simulink model "EMT_load"  (R2024a)
settings: Solver=ode1  StartTime=0.0  StopTime=simtime  FixedStep=Ts  RelTol=1e-3
values from neighbouring files (symbols this model uses):
  c0 = c0_hawk    (= 6.37282e-09)    [EMT_Phasor_parameters.m]
  c1 = c1_hawk    (= 8.76156e-09)    [EMT_Phasor_parameters.m]
  fg = 50    [EMT_Phasor_parameters.m]
  G1gen = 0.1245    [EMT_Phasor_parameters.m]
  G2gen = 0.30    (= 0.3)    [EMT_Phasor_parameters.m]
  G3gen = 0.20    (= 0.2)    [EMT_Phasor_parameters.m]
  G4sgen = 0.2078    [EMT_Phasor_parameters.m]
  G5gen = 0.20    (= 0.2)    [EMT_Phasor_parameters.m]
  G6gen = 0.2078    [EMT_Phasor_parameters.m]
  G6sgen = 0.20    (= 0.2)    [EMT_Phasor_parameters.m]
  G7gen = 0.518    [EMT_Phasor_parameters.m]
  Ihvpk = Ihv*sqrt(2)    [EMT_Phasor_parameters.m]
  l0 = l0_hawk    (= 0.00373)    [EMT_Phasor_parameters.m]
  l1 = l1_hawk    (= 0.00133)    [EMT_Phasor_parameters.m]
  L3dem = 0.10    (= 0.1)    [EMT_Phasor_parameters.m]
  L4dem = 0.30    (= 0.3)    [EMT_Phasor_parameters.m]
  L5dem = 0.35    [EMT_Phasor_parameters.m]
  L6dem = 0.15    [EMT_Phasor_parameters.m]
  L7dem = 0.10    (= 0.1)    [EMT_Phasor_parameters.m]
  Pr = Sr*PF    (= 550050000)    [EMT_Phasor_parameters.m]
  Qr = sqrt(Sr^2 - Pr^2)    [EMT_Phasor_parameters.m]
  r0 = r0_hawk    (= 0.44587)    [EMT_Phasor_parameters.m]
  r1 = r1_hawk    (= 0.12087)    [EMT_Phasor_parameters.m]
  Rtpu = Xtpu/40    (= 0.00375)    [EMT_Phasor_parameters.m]
  S1non = 400e6    (= 400000000)    [EMT_Phasor_parameters.m]
  S2non = 300e6    (= 300000000)    [EMT_Phasor_parameters.m]
  S3non = 200e6    (= 200000000)    [EMT_Phasor_parameters.m]
  S4snon = 200e6    (= 200000000)    [EMT_Phasor_parameters.m]
  S5non = 500e6    (= 500000000)    [EMT_Phasor_parameters.m]
  S6non = 400e6    (= 400000000)    [EMT_Phasor_parameters.m]
  S6snon = 200e6    (= 200000000)    [EMT_Phasor_parameters.m]
  S7non = 200e6    (= 200000000)    [EMT_Phasor_parameters.m]
  simtime = 5    [EMT_Phasor_parameters.m]
  tonvsc = 0.01    [EMT_Phasor_parameters.m]
  Ts = 150e-6    (= 0.00015)    [EMT_Phasor_parameters.m]
  Vhv = 220e3    (= 220000)    [EMT_Phasor_parameters.m]
  Vmv = 22e3    (= 22000)    [EMT_Phasor_parameters.m]
  wc1 = wsw1/10    (= 848.230016469)    [EMT_Phasor_parameters.m]
  wdc1 = wc1/10    (= 84.8230016469)    [EMT_Phasor_parameters.m]
  wpq1 = wc1/10    (= 84.8230016469)    [EMT_Phasor_parameters.m]
  wsw1 = ksw1*2*pi*fg    (= 8482.30016469)    [EMT_Phasor_parameters.m]
  Xtpu = 0.15    [EMT_Phasor_parameters.m]
undefined symbols (not defined in the file or in its folder): D11, Delta, Kf, r, theta0
libraries: simulink_extras x152, spsGroundLib x49, spsCurrentMeasurementLib x39, spsVoltageMeasurementLib x33, simulink x32, eeGeneralControl x32, slpidlib x32, powerlib x30, powerlib_meascontrol x28, spsFirstOrderFilterLib x24, eeTransforms x24, pid_lib x16
(part 5 of 16)

== system EMT_load/G6/VSC/VI measurement ==
  Current Measurement : spsCurrentMeasurementLib/Current Measurement  PhasorSimulation=off  OutputType=Complex  PSBequivalent=0
  Current Measurement1 : spsCurrentMeasurementLib/Current Measurement  PhasorSimulation=off  OutputType=Complex  PSBequivalent=0
  Current Measurement2 : spsCurrentMeasurementLib/Current Measurement  PhasorSimulation=off  OutputType=Complex  PSBequivalent=0
  Ground : spsGroundLib/Ground  LConnTagsString=a
  Ground1 : spsGroundLib/Ground  LConnTagsString=a
  Ground2 : spsGroundLib/Ground  LConnTagsString=a
  Mux : Mux  Inputs=3
  Mux1 : Mux  Inputs=3
  Voltage Measurement : spsVoltageMeasurementLib/Voltage Measurement  PhasorSimulation=off  OutputType=Complex  PSBequivalent=0
  Voltage Measurement1 : spsVoltageMeasurementLib/Voltage Measurement  PhasorSimulation=off  OutputType=Complex  PSBequivalent=0
  Voltage Measurement2 : spsVoltageMeasurementLib/Voltage Measurement  PhasorSimulation=off  OutputType=Complex  PSBequivalent=0
  A : PMIOPort  Side=Left
  B : PMIOPort  Port=2  Side=Left
  C : PMIOPort  Port=3  Side=Left
  a : PMIOPort  Port=4  Side=Right
  b : PMIOPort  Port=5  Side=Right
  c : PMIOPort  Port=6  Side=Right
  Vs : Outport
  Is : Outport  Port=2
  wires:
  Mux1/1 -> Is/1
  Mux/1 -> Vs/1
  Voltage Measurement1/1 -> Mux/2
  Voltage Measurement2/1 -> Mux/3
  Current Measurement2/1 -> Mux1/3
  Voltage Measurement/1 -> Mux/1
  Current Measurement/1 -> Mux1/1
  Current Measurement1/1 -> Mux1/2
  connections:
  Voltage Measurement/LConn1 -- Current Measurement/LConn1 -- A/RConn1
  Current Measurement2/LConn1 -- C/RConn1 -- Voltage Measurement2/LConn1
  Current Measurement1/LConn1 -- Voltage Measurement1/LConn1 -- B/RConn1
  Current Measurement1/RConn1 -- b/RConn1
  Current Measurement/RConn1 -- a/RConn1
  Ground/LConn1 -- Voltage Measurement/LConn2
  Current Measurement2/RConn1 -- c/RConn1
  Ground1/LConn1 -- Voltage Measurement1/LConn2
  Ground2/LConn1 -- Voltage Measurement2/LConn2

== system EMT_load/G6/VSC/VSC Control ==
  Block : Inport
  Vabc : Inport  Port=2
  Iabc : Inport  Port=3
  Pset : Inport  Port=4
  Qset : Inport  Port=5
  Control loops : Subsystem  Variant=on  VariantControlMode=label  LabelModeActiveChoice=EMT_and_QEMT
  Measurements : Subsystem  Variant=on  VariantControlMode=label  LabelModeActiveChoice=EMT
  Modulation : Subsystem  Variant=on  VariantControlMode=label  LabelModeActiveChoice=EMT_AVG
  Mux : Mux  Inputs=2
  Ref : Outport
  m : Outport  Port=2
  wires:
  Control loops/2(iqd+-ref) -> Modulation/3(iqd+-*)
  Control loops/1(vqd+-ref) -> Modulation/2(vqd+-*)
  [PQabc] -> Mux/2
  Measurements/5(PQabc) -> [PQabc]
  Modulation/1(Ref) -> Ref/1
  Measurements/4(theta) -> [theta]
  Vabc/1 -> Measurements/1(Vabc)
  Measurements/1(vqd+-) -> Control loops/3(vqd+-), [vqdpn]
  Measurements/2(iqd+-) -> Control loops/4(iqd+-)
  Measurements/3(freq) -> Control loops/5(freq)
  [theta] -> Modulation/4(theta)
  [vqdpn] -> Modulation/1(vqd+-)
  Iabc/1 -> Measurements/2(Iabc)
  Mux/1 -> m/1
  Control loops/3(m) -> Mux/1
  Pset/1 -> Control loops/1(Pset)
  Qset/1 -> Control loops/2(Qset)
  Block/1 -> Control loops/6(Block)

== system EMT_load/G6/VSC/VSC Model ==
  Ref : Inport
  EMT AVG : Subsystem  VariantControl=EMT_AVG
      settings: PortSchema="{\"entries\":[{\"content\":{\"sides\":[{\"content\":{\"connectorIds\":[\"LConn1\",\"LConn2\",\"LConn3\"]},\"type\":\"ConnectorPlacement.EquallySpacedRectSide\",\"uuid\":\"96043b84-a665-4cb2-a938-d6633d7ee474\"},{\"content\":{\"connectorIds\":[\"In1\"],\"side\":\"RIGHT\"},\"type\":\"ConnectorPlacement.EquallySpacedRectSide\",\"uuid\":\"064d463f-c23a-42ac-89ce-8dea3d446214\"},{\"content\":{\"connectorIds\":[],\"side\":\"TOP\"},\"type\":\"ConnectorPlacement.EquallySpacedRectSide\",\"uuid\":\"95ef669c-c6ed-44c3-8b69-447906728b6d\"}]},\"type\":\"ConnectorPlacement.EquallySpacedConnector\",\"uuid\":\"ea66db09-64d7-4d7e-ba7b-d769c56e2dbd\"}],\"packageUris\":[\"http://schema.mathworks.com/mf0/Connector/19700101\"],\"version\":\"1.0\"}"
  EMT SW : Subsystem  VariantControl=EMT_SW
      settings: PortSchema="{\"entries\":[{\"content\":{\"sides\":[{\"content\":{\"connectorIds\":[\"LConn1\",\"LConn2\",\"LConn3\"]},\"type\":\"ConnectorPlacement.EquallySpacedRectSide\",\"uuid\":\"96043b84-a665-4cb2-a938-d6633d7ee474\"},{\"content\":{\"connectorIds\":[\"In1\"],\"side\":\"RIGHT\"},\"type\":\"ConnectorPlacement.EquallySpacedRectSide\",\"uuid\":\"064d463f-c23a-42ac-89ce-8dea3d446214\"},{\"content\":{\"connectorIds\":[],\"side\":\"TOP\"},\"type\":\"ConnectorPlacement.EquallySpacedRectSide\",\"uuid\":\"95ef669c-c6ed-44c3-8b69-447906728b6d\"}]},\"type\":\"ConnectorPlacement.EquallySpacedConnector\",\"uuid\":\"ea66db09-64d7-4d7e-ba7b-d769c56e2dbd\"}],\"packageUris\":[\"http://schema.mathworks.com/mf0/Connector/19700101\"],\"version\":\"1.0\"}"
  Phasor : Subsystem  VariantControl=Phasor
      settings: PortSchema="{\"entries\":[{\"content\":{\"sides\":[{\"content\":{\"connectorIds\":[\"LConn1\",\"LConn2\",\"LConn3\"]},\"type\":\"ConnectorPlacement.EquallySpacedRectSide\",\"uuid\":\"96043b84-a665-4cb2-a938-d6633d7ee474\"},{\"content\":{\"connectorIds\":[\"In1\"],\"side\":\"RIGHT\"},\"type\":\"ConnectorPlacement.EquallySpacedRectSide\",\"uuid\":\"064d463f-c23a-42ac-89ce-8dea3d446214\"},{\"content\":{\"connectorIds\":[],\"side\":\"TOP\"},\"type\":\"ConnectorPlacement.EquallySpacedRectSide\",\"uuid\":\"95ef669c-c6ed-44c3-8b69-447906728b6d\"}]},\"type\":\"ConnectorPlacement.EquallySpacedConnector\",\"uuid\":\"ea66db09-64d7-4d7e-ba7b-d769c56e2dbd\"}],\"packageUris\":[\"http://schema.mathworks.com/mf0/Connector/19700101\"],\"version\":\"1.0\"}"
  A : PMIOPort  Side=Left
  B : PMIOPort  Port=2  Side=Left
  C : PMIOPort  Port=3  Side=Left

== system EMT_load/G6/VSC/output signals ==
  Vs : Inport
  Is : Inport  Port=2
  control : Inport  Port=3
  Bus Creator : BusCreator  Inputs=15
  Demux : Demux  Outputs=13
  m : Outport
  wires:
  Bus Creator/1 -> m/1
  control/1 -> Demux/1
  Vs/1 -> Bus Creator/1  "Vabc"
  Is/1 -> Bus Creator/2  "Iabc"
  Demux/1 -> Bus Creator/3  "vqp"
  Demux/2 -> Bus Creator/4  "vdp"
  Demux/3 -> Bus Creator/5  "vqn"
  Demux/4 -> Bus Creator/6  "vdn"
  Demux/5 -> Bus Creator/7  "iqp"
  Demux/6 -> Bus Creator/8  "idp"
  Demux/7 -> Bus Creator/9  "iqn"
  Demux/8 -> Bus Creator/10  "idn"
  Demux/9 -> Bus Creator/11  "f"
  Demux/10 -> Bus Creator/12  "Pdq"
  Demux/11 -> Bus Creator/13  "Qdq"
  Demux/12 -> Bus Creator/14  "Pabc"
  Demux/13 -> Bus Creator/15  "Qabc"

== system EMT_load/G6s/Exciter System/PSS ==
  note: Power System Stabilizer (PSS2A)
  dw : Inport
  Pgen : Inport  Port=2
  Gain : Gain  Gain=Ks1
  Gain1 : Gain  Gain=Ks3
  Saturation : Saturate  UpperLimit=Vstmax  LowerLimit=Vstmin
  Sum1 : Sum  Inputs=|++
  Sum2 : Sum  Inputs=|+-
  Transfer Fcn1 : TransferFcn  Numerator=[Tw1 0]  Denominator=[Tw1 1]
  Transfer Fcn2 : TransferFcn  Numerator=[Tw3 0]  Denominator=[Tw3 1]
  Transfer Fcn3 : TransferFcn  Numerator=[Tw2 0]  Denominator=[Tw2 1]
  Transfer Fcn4 : TransferFcn  Denominator=[T6 1]
  Transfer Fcn5 : TransferFcn  Numerator=[T8 1].^N  Denominator=[T9 1].^(M*N)
  Transfer Fcn6 : TransferFcn  Numerator=[T1 1]  Denominator=[T2 1]
  Transfer Fcn7 : TransferFcn  Numerator=[T3 1]  Denominator=[T4 1]
  Transfer Fcn8 : TransferFcn  Numerator=[Tw4 0]  Denominator=[Tw4 1]
  Transfer Fcn9 : TransferFcn  Numerator=[Ks2]  Denominator=[T7 1]
  Vothsg : Outport
  wires:
  Transfer Fcn9/1 -> Sum2/2, Gain1/1
  Gain1/1 -> Sum1/2
  Transfer Fcn8/1 -> Transfer Fcn9/1
  Transfer Fcn2/1 -> Transfer Fcn8/1
  Pgen/1 -> Transfer Fcn2/1
  Saturation/1 -> Vothsg/1
  Transfer Fcn7/1 -> Saturation/1
  Transfer Fcn6/1 -> Transfer Fcn7/1
  Gain/1 -> Transfer Fcn6/1
  Sum2/1 -> Gain/1
  Transfer Fcn5/1 -> Sum2/1
  Sum1/1 -> Transfer Fcn5/1
  Transfer Fcn4/1 -> Sum1/1
  Transfer Fcn3/1 -> Transfer Fcn4/1
  Transfer Fcn1/1 -> Transfer Fcn3/1
  dw/1 -> Transfer Fcn1/1

== system EMT_load/G6s/Exciter System/SEXS ==
  note: The controller parameters provided by ENTSO-E
      | define different names for the parameters:
      |
      | ENTSO-E = IEEE Std 421.5-2005
      | Ta = Tc
      | Tb = Tb
      | K = Ka
      | Te = Ta
      | Emax = Vrmax
      | Emin = Vrmin
  note: The exciter model provided by ENTSO-E most similar to the IEEE is the Type AC4A excitation system model
  Vref : Inport
  Vc : Inport  Port=2
  Vs : Inport  Port=3
  1st ord transfer fcn windup limiter : Subsystem  mask{Gain=K, tau=Te, Vmax=Emax, Vmin=Emin, y0=Vf0}
      mask prompts: tau "Time constant"; y0 "Initial output"
  Constant : Constant  Value=Vf0/K
  Saturation : Saturate  Commented=through  UpperLimit=0.1  LowerLimit=-0.1
  Sum : Sum  Inputs=+-+
  Sum1 : Sum  Inputs=|++
  Transfer Fcn (with initial outputs)1 : simulink_extras/Additional Linear/Transfer Fcn (with initial outputs)  N=[Ta 1]  D=[Tb 1]  Y0=Vf0/K  U0=Vf0/K
  Efd : Outport
  wires:
  1st ord transfer fcn windup limiter/1(Out1) -> Efd/1
  Vs/1 -> Sum/3
  Vref/1 -> Sum/1
  Vc/1 -> Sum/2
  Transfer Fcn (with initial outputs)1/1 -> 1st ord transfer fcn windup limiter/1(In1)
  Saturation/1 -> Transfer Fcn (with initial outputs)1/1
  Sum/1 -> Sum1/1
  Sum1/1 -> Saturation/1
  Constant/1 -> Sum1/2

== system EMT_load/G6s/Exciter System/TR and LC_test ==
  note: Rc and Xc should be negative values in case of voltage regulated after an impedance
  note: Fig 4.1 of IEEE Std 421.5-2005
  note: Vt and It should be phasors (complex quantities)
  note: compensated
      | impedance
  note: Terminal voltage transducer and optional load compensation
  Vt : Inport
  It : Inport  Port=2
  Abs : Abs  SaturateOnIntegerOverflow=off
  Abs1 : Abs  SaturateOnIntegerOverflow=off
  Rc+jXc : Gain  Gain=abs(Rc+1i*Xc)
  Saturation : Saturate  UpperLimit=1.2  LowerLimit=0.8
  Sum : Sum  Inputs=|+-
  Transfer Fcn (with initial outputs) : simulink_extras/Additional Linear/Transfer Fcn (with initial outputs)  N=[1]  D=[Tr 1]  Y0=1  U0=1
  Vc : Outport
  wires:
  Abs1/1 -> Rc+jXc/1
  Abs/1 -> Sum/1
  It/1 -> Abs1/1
  Sum/1 -> Transfer Fcn (with initial outputs)/1
  Rc+jXc/1 -> Sum/2
  Transfer Fcn (with initial outputs)/1 -> Saturation/1
  Vt/1 -> Abs/1
  Saturation/1 -> Vc/1

== system EMT_load/G7/Exciter System/PSS1 ==
  note: Power System Stabilizer (PSS2A)
  dw : Inport
  Pgen : Inport  Port=2
  Gain : Gain  Gain=Ks1
  Gain1 : Gain  Gain=Ks3
  Saturation : Saturate  UpperLimit=Vstmax  LowerLimit=Vstmin
  Sum1 : Sum  Inputs=|++
  Sum2 : Sum  Inputs=|+-
  Transfer Fcn1 : TransferFcn  Numerator=[Tw1 0]  Denominator=[Tw1 1]
  Transfer Fcn2 : TransferFcn  Numerator=[Tw3 0]  Denominator=[Tw3 1]
  Transfer Fcn3 : TransferFcn  Numerator=[Tw2 0]  Denominator=[Tw2 1]
  Transfer Fcn4 : TransferFcn  Denominator=[T6 1]
  Transfer Fcn5 : TransferFcn  Numerator=[T8 1].^N  Denominator=[T9 1].^(M*N)
  Transfer Fcn6 : TransferFcn  Numerator=[T1 1]  Denominator=[T2 1]
  Transfer Fcn7 : TransferFcn  Numerator=[T3 1]  Denominator=[T4 1]
  Transfer Fcn8 : TransferFcn  Numerator=[Tw4 0]  Denominator=[Tw4 1]
  Transfer Fcn9 : TransferFcn  Numerator=[Ks2]  Denominator=[T7 1]
  Vothsg : Outport
  wires:
  dw/1 -> Transfer Fcn1/1
  Transfer Fcn1/1 -> Transfer Fcn3/1
  Transfer Fcn3/1 -> Transfer Fcn4/1
  Transfer Fcn4/1 -> Sum1/1
  Sum1/1 -> Transfer Fcn5/1
  Transfer Fcn5/1 -> Sum2/1
  Sum2/1 -> Gain/1
  Gain/1 -> Transfer Fcn6/1
  Transfer Fcn6/1 -> Transfer Fcn7/1
  Transfer Fcn7/1 -> Saturation/1
  Saturation/1 -> Vothsg/1
  Pgen/1 -> Transfer Fcn2/1
  Transfer Fcn2/1 -> Transfer Fcn8/1
  Transfer Fcn8/1 -> Transfer Fcn9/1
  Gain1/1 -> Sum1/2
  Transfer Fcn9/1 -> Gain1/1, Sum2/2

== system EMT_load/G7/Exciter System/SEXS ==
  note: The controller parameters provided by ENTSO-E
      | define different names for the parameters:
      |
      | ENTSO-E = IEEE Std 421.5-2005
      | Ta = Tc
      | Tb = Tb
      | K = Ka
      | Te = Ta
      | Emax = Vrmax
      | Emin = Vrmin
  note: The exciter model provided by ENTSO-E most similar to the IEEE is the Type AC4A excitation system model
  Vref : Inport
  Vc : Inport  Port=2
  Vs : Inport  Port=3
  1st ord transfer fcn windup limiter : Subsystem  mask{Gain=K, tau=Te, Vmax=Emax, Vmin=Emin, y0=Vf0}
      mask prompts: tau "Time constant"; y0 "Initial output"
  Constant : Constant  Value=Vf0/K
  Saturation : Saturate  Commented=through  UpperLimit=0.1  LowerLimit=-0.1
  Sum : Sum  Inputs=+-+
  Sum1 : Sum  Inputs=|++
  Transfer Fcn (with initial outputs)1 : simulink_extras/Additional Linear/Transfer Fcn (with initial outputs)  N=[Ta 1]  D=[Tb 1]  Y0=Vf0/K  U0=Vf0/K
  Efd : Outport
  wires:
  1st ord transfer fcn windup limiter/1(Out1) -> Efd/1
  Vs/1 -> Sum/3
  Vref/1 -> Sum/1
  Vc/1 -> Sum/2
  Transfer Fcn (with initial outputs)1/1 -> 1st ord transfer fcn windup limiter/1(In1)
  Saturation/1 -> Transfer Fcn (with initial outputs)1/1
  Sum/1 -> Sum1/1
  Sum1/1 -> Saturation/1
  Constant/1 -> Sum1/2

== system EMT_load/G7/Exciter System/TR and LC_test ==
  note: Terminal voltage transducer and optional load compensation
  note: compensated
      | impedance
  note: Vt and It should be phasors (complex quantities)
  note: Fig 4.1 of IEEE Std 421.5-2005
  note: Rc and Xc should be negative values in case of voltage regulated after an impedance
  Vt : Inport
  It : Inport  Port=2
  Abs : Abs  SaturateOnIntegerOverflow=off
  Abs1 : Abs  SaturateOnIntegerOverflow=off
  Rc+jXc : Gain  Gain=abs(Rc+1i*Xc)
  Saturation : Saturate  UpperLimit=1.2  LowerLimit=0.8
  Sum : Sum  Inputs=|+-
  Transfer Fcn (with initial outputs) : simulink_extras/Additional Linear/Transfer Fcn (with initial outputs)  Commented=through  N=[1]  D=[Tr 1]  Y0=1  U0=1
  Vc : Outport
  wires:
  Saturation/1 -> Vc/1
  Vt/1 -> Abs/1
  Transfer Fcn (with initial outputs)/1 -> Saturation/1
  Rc+jXc/1 -> Sum/2
  Sum/1 -> Transfer Fcn (with initial outputs)/1
  It/1 -> Abs1/1
  Abs/1 -> Sum/1
  Abs1/1 -> Rc+jXc/1

== system EMT_load/G1/Exciter System/SEXS/1st ord transfer fcn windup limiter ==
  note: First order transfer function with windup limiter (non-saturated output)
  In1 : Inport
  Compare To Constant : simulink/Logic and Bit Operations/Compare To Constant  relop=<=  const=Vmax  OutDataTypeStr=boolean
  Compare To Constant1 : simulink/Logic and Bit Operations/Compare To Constant  relop=>=  const=Vmin  OutDataTypeStr=boolean
  OR : Logic  Operator=OR  IconShape=distinctive  AllPortsSameDT=off  OutDataTypeStr=boolean
  Sample and Hold1 : spsSampleandHoldLib/Sample and Hold  ic=0  Ts=0
      settings: LibrarySourceBlock=|
      | sps_lib/Control/Sample and
      | Hold
  Saturation1 : Saturate  UpperLimit=Vmax  LowerLimit=Vmin
  Transfer Fcn (with initial outputs)2 : simulink_extras/Additional Linear/Transfer Fcn (with initial outputs)  N=[Gain]  D=[tau 1]  Y0=y0  U0=y0/Gain
  Out1 : Outport
  wires:
  Sample and Hold1/1 -> Transfer Fcn (with initial outputs)2/1
  Transfer Fcn (with initial outputs)2/1 -> Saturation1/1, Compare To Constant1/1, Compare To Constant/1
  In1/1 -> Sample and Hold1/1
  Compare To Constant/1 -> OR/1
  Compare To Constant1/1 -> OR/2
  OR/1 -> Sample and Hold1/2
  Saturation1/1 -> Out1/1

== system EMT_load/G2/VSC/VSC Control/Control loops ==
  note: 1) Add Subsystem or Model blocks as valid variant choices.
      | 2) You cannot connect blocks at this level. At simulation, connectivity is automatically
      | determined, based on the active variant and port name matching.
  Pset : Inport
  Qset : Inport  Port=2
  vqd+- : Inport  Port=3
  iqd+- : Inport  Port=4
  freq : Inport  Port=5
  Block : Inport  Port=6
  Phasor I 1st : Subsystem  VariantControl=Phasor_I_1st
  Phasor I ref : Subsystem  VariantControl=Phasor_I_ref
  Phasor PQ 1st : Subsystem  VariantControl=Phasor_PQ
  "SW, EMT AVG, Phasor Quasi-EMT" : Subsystem  VariantControl=EMT_and_QEMT
  vqd+-ref : Outport
  iqd+-ref : Outport  Port=2
  m : Outport  Port=3

== system EMT_load/G2/VSC/VSC Control/Measurements ==
  note: 1) Add Subsystem or Model blocks as valid variant choices.
      | 2) You cannot connect blocks at this level. At simulation, connectivity is automatically
      | determined, based on the active variant and port name matching.
  Vabc : Inport
  Iabc : Inport  Port=2
  EMT : Subsystem  VariantControl=EMT
  Phasor : Subsystem  VariantControl=Phasor
  vqd+- : Outport
  iqd+- : Outport  Port=2
  freq : Outport  Port=3
  theta : Outport  Port=4
  PQabc : Outport  Port=5

== system EMT_load/G2/VSC/VSC Control/Modulation ==
  note: 1) Add Subsystem or Model blocks as valid variant choices.
      | 2) You cannot connect blocks at this level. At simulation, connectivity is automatically
      | determined, based on the active variant and port name matching.
  vqd+- : Inport
  vqd+-* : Inport  Port=2
  iqd+-* : Inport  Port=3
  theta : Inport  Port=4
  EMT AVG : Subsystem  VariantControl=EMT_AVG
  EMT Switching : Subsystem  VariantControl=EMT_SW
  Phasor I and Phasor PQ : Subsystem  VariantControl=Phasor_I_and_PQ
  Phasor Quasi-EMT : Subsystem  VariantControl=Phasor_QEMT
  Ref : Outport

== system EMT_load/G2/VSC/VSC Model/EMT AVG ==
  Ref : Inport
  Controlled Voltage Source3 : spsControlledVoltageSourceLib/Controlled Voltage Source  Initialize=off  Source_Type=AC  Amplitude=Vhvpk  Phase=0  Frequency=fg  Measurements=None
  Controlled Voltage Source4 : spsControlledVoltageSourceLib/Controlled Voltage Source  Initialize=off  Source_Type=AC  Amplitude=Vhvpk  Phase=-2*pi/3  Frequency=fg  Measurements=None
  Controlled Voltage Source5 : spsControlledVoltageSourceLib/Controlled Voltage Source  Initialize=off  Source_Type=AC  Amplitude=Vhvpk  Phase=-4*pi/3  Frequency=fg  Measurements=None
  Demux1 : Demux  Outputs=3
  Ground : spsGroundLib/Ground  LConnTagsString=a
  Ground4 : spsGroundLib/Ground  LConnTagsString=a
  Ground5 : spsGroundLib/Ground  LConnTagsString=a
  A : PMIOPort  Side=Left
  B : PMIOPort  Port=2  Side=Left
  C : PMIOPort  Port=3  Side=Left
  wires:
  Ref/1 -> Demux1/1
  Demux1/1 -> Controlled Voltage Source3/1
  Demux1/2 -> Controlled Voltage Source4/1
  Demux1/3 -> Controlled Voltage Source5/1
  connections:
  Controlled Voltage Source3/RConn1 -- A/RConn1
  Controlled Voltage Source4/RConn1 -- B/RConn1
  Controlled Voltage Source5/RConn1 -- C/RConn1
  Ground/LConn1 -- Controlled Voltage Source3/LConn1
  Ground4/LConn1 -- Controlled Voltage Source4/LConn1
  Ground5/LConn1 -- Controlled Voltage Source5/LConn1

== system EMT_load/G2/VSC/VSC Model/EMT SW ==
  Ref : Inport
  DC Voltage Source : powerlib/Electrical Sources/DC Voltage Source  Amplitude=Vdc  Measurements=None
  Universal Bridge : powerlib/Power Electronics/Universal Bridge  Arms=3  SnubberResistance=1e6  SnubberCapacitance=inf  Device=IGBT / Diodes  Ron=1e-4  Lon=0  ForwardVoltages="[  0  0  ]"  ForwardVoltage=0  GTOparameters=[ 10e-6 , 20e-6 ]  IGBTparameters=[ 1e-6 , 2e-6 ]  Measurements=None  Measurements_2=None  converterType=Rectifier
  A : PMIOPort  Side=Left
  B : PMIOPort  Port=2  Side=Left
  C : PMIOPort  Port=3  Side=Left
  wires:
  Ref/1 -> Universal Bridge/1
  connections:
  Universal Bridge/LConn2 -- B/RConn1
  Universal Bridge/LConn1 -- A/RConn1
  Universal Bridge/LConn3 -- C/RConn1
  Universal Bridge/RConn1 -- DC Voltage Source/RConn1
  Universal Bridge/RConn2 -- DC Voltage Source/LConn1

== system EMT_load/G2/VSC/VSC Model/Phasor ==
  Ref : Inport
  Controlled Current Source : powerlib/Electrical Sources/Controlled Current Source  Initialize=off  Source_Type=AC  Amplitude=0  Phase=0  Frequency=0  Measurements=None
  Controlled Current Source1 : powerlib/Electrical Sources/Controlled Current Source  Initialize=off  Source_Type=AC  Amplitude=0  Phase=0  Frequency=0  Measurements=None
  Controlled Current Source2 : powerlib/Electrical Sources/Controlled Current Source  Initialize=off  Source_Type=AC  Amplitude=0  Phase=0  Frequency=0  Measurements=None
  Demux1 : Demux  Outputs=3
  Ground{1..3,5} (4 alike) : powerlib/Elements/Ground  LConnTagsString=a
  Three-Phase Series RLC Branch : powerlib/Elements/Three-Phase Series RLC Branch  LConnTagsString=A|B|C  RConnTagsString=A|B|C  BranchType=R  Resistance=1e7  Inductance=1e-3  Capacitance=1e-6  Measurements=None
  A : PMIOPort  Side=Left
  B : PMIOPort  Port=2  Side=Left
  C : PMIOPort  Port=3  Side=Left
  wires:
  [c] -> Controlled Current Source2/1
  [b] -> Controlled Current Source1/1
  [a] -> Controlled Current Source/1
  Demux1/3 -> [c]
  Demux1/2 -> [b]
  Demux1/1 -> [a]
  Ref/1 -> Demux1/1
  connections:
  Controlled Current Source/RConn1 -- Ground1/LConn1
  Controlled Current Source1/RConn1 -- Ground2/LConn1
  Controlled Current Source2/RConn1 -- Ground3/LConn1
  A/RConn1 -- Controlled Current Source/LConn1 -- Three-Phase Series RLC Branch/LConn1
  C/RConn1 -- Controlled Current Source2/LConn1 -- Three-Phase Series RLC Branch/LConn3
  Ground5/LConn1 -- Three-Phase Series RLC Branch/RConn2 -- Three-Phase Series RLC Branch/RConn1 -- Three-Phase Series RLC Branch/RConn3
  Controlled Current Source1/LConn1 -- Three-Phase Series RLC Branch/LConn2 -- B/RConn1

== system EMT_load/G3/VSC/VSC Control/Control loops ==
  note: 1) Add Subsystem or Model blocks as valid variant choices.
      | 2) You cannot connect blocks at this level. At simulation, connectivity is automatically
      | determined, based on the active variant and port name matching.
  Pset : Inport
  Qset : Inport  Port=2
  vqd+- : Inport  Port=3
  iqd+- : Inport  Port=4
  freq : Inport  Port=5
  Block : Inport  Port=6
  Phasor I 1st : Subsystem  VariantControl=Phasor_I_1st
  Phasor I ref : Subsystem  VariantControl=Phasor_I_ref
  Phasor PQ 1st : Subsystem  VariantControl=Phasor_PQ
  "SW, EMT AVG, Phasor Quasi-EMT" : Subsystem  VariantControl=EMT_and_QEMT
  vqd+-ref : Outport
  iqd+-ref : Outport  Port=2
  m : Outport  Port=3

== system EMT_load/G3/VSC/VSC Control/Measurements ==
  note: 1) Add Subsystem or Model blocks as valid variant choices.
      | 2) You cannot connect blocks at this level. At simulation, connectivity is automatically
      | determined, based on the active variant and port name matching.
  Vabc : Inport
  Iabc : Inport  Port=2
  EMT : Subsystem  VariantControl=EMT
  Phasor : Subsystem  VariantControl=Phasor
  vqd+- : Outport
  iqd+- : Outport  Port=2
  freq : Outport  Port=3
  theta : Outport  Port=4
  PQabc : Outport  Port=5

== system EMT_load/G3/VSC/VSC Control/Modulation ==
  note: 1) Add Subsystem or Model blocks as valid variant choices.
      | 2) You cannot connect blocks at this level. At simulation, connectivity is automatically
      | determined, based on the active variant and port name matching.
  vqd+- : Inport
  vqd+-* : Inport  Port=2
  iqd+-* : Inport  Port=3
  theta : Inport  Port=4
  EMT AVG : Subsystem  VariantControl=EMT_AVG
  EMT Switching : Subsystem  VariantControl=EMT_SW
  Phasor I and Phasor PQ : Subsystem  VariantControl=Phasor_I_and_PQ
  Phasor Quasi-EMT : Subsystem  VariantControl=Phasor_QEMT
  Ref : Outport

== system EMT_load/G3/VSC/VSC Model/EMT AVG ==
  Ref : Inport
  Controlled Voltage Source3 : spsControlledVoltageSourceLib/Controlled Voltage Source  Initialize=off  Source_Type=AC  Amplitude=Vhvpk  Phase=0  Frequency=fg  Measurements=None
  Controlled Voltage Source4 : spsControlledVoltageSourceLib/Controlled Voltage Source  Initialize=off  Source_Type=AC  Amplitude=Vhvpk  Phase=-2*pi/3  Frequency=fg  Measurements=None
  Controlled Voltage Source5 : spsControlledVoltageSourceLib/Controlled Voltage Source  Initialize=off  Source_Type=AC  Amplitude=Vhvpk  Phase=-4*pi/3  Frequency=fg  Measurements=None
  Demux1 : Demux  Outputs=3
  Ground : spsGroundLib/Ground  LConnTagsString=a
  Ground4 : spsGroundLib/Ground  LConnTagsString=a
  Ground5 : spsGroundLib/Ground  LConnTagsString=a
  A : PMIOPort  Side=Left
  B : PMIOPort  Port=2  Side=Left
  C : PMIOPort  Port=3  Side=Left
  wires:
  Ref/1 -> Demux1/1
  Demux1/1 -> Controlled Voltage Source3/1
  Demux1/2 -> Controlled Voltage Source4/1
  Demux1/3 -> Controlled Voltage Source5/1
  connections:
  Controlled Voltage Source3/RConn1 -- A/RConn1
  Controlled Voltage Source4/RConn1 -- B/RConn1
  Controlled Voltage Source5/RConn1 -- C/RConn1
  Ground/LConn1 -- Controlled Voltage Source3/LConn1
  Ground4/LConn1 -- Controlled Voltage Source4/LConn1
  Ground5/LConn1 -- Controlled Voltage Source5/LConn1

== system EMT_load/G3/VSC/VSC Model/EMT SW ==
  Ref : Inport
  DC Voltage Source : powerlib/Electrical Sources/DC Voltage Source  Amplitude=Vdc  Measurements=None
  Universal Bridge : powerlib/Power Electronics/Universal Bridge  Arms=3  SnubberResistance=1e6  SnubberCapacitance=inf  Device=IGBT / Diodes  Ron=1e-4  Lon=0  ForwardVoltages="[  0  0  ]"  ForwardVoltage=0  GTOparameters=[ 10e-6 , 20e-6 ]  IGBTparameters=[ 1e-6 , 2e-6 ]  Measurements=None  Measurements_2=None  converterType=Rectifier
  A : PMIOPort  Side=Left
  B : PMIOPort  Port=2  Side=Left
  C : PMIOPort  Port=3  Side=Left
  wires:
  Ref/1 -> Universal Bridge/1
  connections:
  Universal Bridge/LConn2 -- B/RConn1
  Universal Bridge/LConn1 -- A/RConn1
  Universal Bridge/LConn3 -- C/RConn1
  Universal Bridge/RConn1 -- DC Voltage Source/RConn1
  Universal Bridge/RConn2 -- DC Voltage Source/LConn1

== system EMT_load/G3/VSC/VSC Model/Phasor ==
  Ref : Inport
  Controlled Current Source : powerlib/Electrical Sources/Controlled Current Source  Initialize=off  Source_Type=AC  Amplitude=0  Phase=0  Frequency=0  Measurements=None
  Controlled Current Source1 : powerlib/Electrical Sources/Controlled Current Source  Initialize=off  Source_Type=AC  Amplitude=0  Phase=0  Frequency=0  Measurements=None
  Controlled Current Source2 : powerlib/Electrical Sources/Controlled Current Source  Initialize=off  Source_Type=AC  Amplitude=0  Phase=0  Frequency=0  Measurements=None
  Demux1 : Demux  Outputs=3
  Ground{1..3,5} (4 alike) : powerlib/Elements/Ground  LConnTagsString=a
  Three-Phase Series RLC Branch : powerlib/Elements/Three-Phase Series RLC Branch  LConnTagsString=A|B|C  RConnTagsString=A|B|C  BranchType=R  Resistance=1e7  Inductance=1e-3  Capacitance=1e-6  Measurements=None
  A : PMIOPort  Side=Left
  B : PMIOPort  Port=2  Side=Left
  C : PMIOPort  Port=3  Side=Left
  wires:
  [c] -> Controlled Current Source2/1
  [b] -> Controlled Current Source1/1
  [a] -> Controlled Current Source/1
  Demux1/3 -> [c]
  Demux1/2 -> [b]
  Demux1/1 -> [a]
  Ref/1 -> Demux1/1
  connections:
  Controlled Current Source/RConn1 -- Ground1/LConn1
  Controlled Current Source1/RConn1 -- Ground2/LConn1
  Controlled Current Source2/RConn1 -- Ground3/LConn1
  A/RConn1 -- Controlled Current Source/LConn1 -- Three-Phase Series RLC Branch/LConn1
  C/RConn1 -- Controlled Current Source2/LConn1 -- Three-Phase Series RLC Branch/LConn3
  Ground5/LConn1 -- Three-Phase Series RLC Branch/RConn2 -- Three-Phase Series RLC Branch/RConn1 -- Three-Phase Series RLC Branch/RConn3
  Controlled Current Source1/LConn1 -- Three-Phase Series RLC Branch/LConn2 -- B/RConn1

== system EMT_load/G4s/Exciter System/SEXS/1st ord transfer fcn windup limiter ==
  note: First order transfer function with windup limiter (non-saturated output)
  In1 : Inport
  Compare To Constant : simulink/Logic and Bit Operations/Compare To Constant  relop=<=  const=Vmax  OutDataTypeStr=boolean
  Compare To Constant1 : simulink/Logic and Bit Operations/Compare To Constant  relop=>=  const=Vmin  OutDataTypeStr=boolean
  OR : Logic  Operator=OR  IconShape=distinctive  AllPortsSameDT=off  OutDataTypeStr=boolean
  Sample and Hold1 : spsSampleandHoldLib/Sample and Hold  ic=0  Ts=0
      settings: LibrarySourceBlock=|
      | sps_lib/Control/Sample and
      | Hold
  Saturation1 : Saturate  UpperLimit=Vmax  LowerLimit=Vmin
  Transfer Fcn (with initial outputs)2 : simulink_extras/Additional Linear/Transfer Fcn (with initial outputs)  N=[Gain]  D=[tau 1]  Y0=y0  U0=y0/Gain
  Out1 : Outport
  wires:
  Sample and Hold1/1 -> Transfer Fcn (with initial outputs)2/1
  Transfer Fcn (with initial outputs)2/1 -> Saturation1/1, Compare To Constant1/1, Compare To Constant/1
  In1/1 -> Sample and Hold1/1
  Compare To Constant/1 -> OR/1
  Compare To Constant1/1 -> OR/2
  OR/1 -> Sample and Hold1/2
  Saturation1/1 -> Out1/1

== system EMT_load/G5/VSC/VSC Control/Control loops ==
  note: 1) Add Subsystem or Model blocks as valid variant choices.
      | 2) You cannot connect blocks at this level. At simulation, connectivity is automatically
      | determined, based on the active variant and port name matching.
  Pset : Inport
  Qset : Inport  Port=2
  vqd+- : Inport  Port=3
  iqd+- : Inport  Port=4
  freq : Inport  Port=5
  Block : Inport  Port=6
  Phasor I 1st : Subsystem  VariantControl=Phasor_I_1st
  Phasor I ref : Subsystem  VariantControl=Phasor_I_ref
  Phasor PQ 1st : Subsystem  VariantControl=Phasor_PQ
  "SW, EMT AVG, Phasor Quasi-EMT" : Subsystem  VariantControl=EMT_and_QEMT
  vqd+-ref : Outport
  iqd+-ref : Outport  Port=2
  m : Outport  Port=3

== system EMT_load/G5/VSC/VSC Control/Measurements ==
  note: 1) Add Subsystem or Model blocks as valid variant choices.
      | 2) You cannot connect blocks at this level. At simulation, connectivity is automatically
      | determined, based on the active variant and port name matching.
  Vabc : Inport
  Iabc : Inport  Port=2
  EMT : Subsystem  VariantControl=EMT
  Phasor : Subsystem  VariantControl=Phasor
  vqd+- : Outport
  iqd+- : Outport  Port=2
  freq : Outport  Port=3
  theta : Outport  Port=4
  PQabc : Outport  Port=5

== system EMT_load/G5/VSC/VSC Control/Modulation ==
  note: 1) Add Subsystem or Model blocks as valid variant choices.
      | 2) You cannot connect blocks at this level. At simulation, connectivity is automatically
      | determined, based on the active variant and port name matching.
  vqd+- : Inport
  vqd+-* : Inport  Port=2
  iqd+-* : Inport  Port=3
  theta : Inport  Port=4
  EMT AVG : Subsystem  VariantControl=EMT_AVG
  EMT Switching : Subsystem  VariantControl=EMT_SW
  Phasor I and Phasor PQ : Subsystem  VariantControl=Phasor_I_and_PQ
  Phasor Quasi-EMT : Subsystem  VariantControl=Phasor_QEMT
  Ref : Outport

== system EMT_load/G5/VSC/VSC Model/EMT AVG ==
  Ref : Inport
  Controlled Voltage Source3 : spsControlledVoltageSourceLib/Controlled Voltage Source  Initialize=off  Source_Type=AC  Amplitude=Vhvpk  Phase=0  Frequency=fg  Measurements=None
  Controlled Voltage Source4 : spsControlledVoltageSourceLib/Controlled Voltage Source  Initialize=off  Source_Type=AC  Amplitude=Vhvpk  Phase=-2*pi/3  Frequency=fg  Measurements=None
  Controlled Voltage Source5 : spsControlledVoltageSourceLib/Controlled Voltage Source  Initialize=off  Source_Type=AC  Amplitude=Vhvpk  Phase=-4*pi/3  Frequency=fg  Measurements=None
  Demux1 : Demux  Outputs=3
  Ground : spsGroundLib/Ground  LConnTagsString=a
  Ground4 : spsGroundLib/Ground  LConnTagsString=a
  Ground5 : spsGroundLib/Ground  LConnTagsString=a
  A : PMIOPort  Side=Left
  B : PMIOPort  Port=2  Side=Left
  C : PMIOPort  Port=3  Side=Left
  wires:
  Ref/1 -> Demux1/1
  Demux1/1 -> Controlled Voltage Source3/1
  Demux1/2 -> Controlled Voltage Source4/1
  Demux1/3 -> Controlled Voltage Source5/1
  connections:
  Controlled Voltage Source3/RConn1 -- A/RConn1
  Controlled Voltage Source4/RConn1 -- B/RConn1
  Controlled Voltage Source5/RConn1 -- C/RConn1
  Ground/LConn1 -- Controlled Voltage Source3/LConn1
  Ground4/LConn1 -- Controlled Voltage Source4/LConn1
  Ground5/LConn1 -- Controlled Voltage Source5/LConn1

== system EMT_load/G5/VSC/VSC Model/EMT SW ==
  Ref : Inport
  DC Voltage Source : powerlib/Electrical Sources/DC Voltage Source  Amplitude=Vdc  Measurements=None
  Universal Bridge : powerlib/Power Electronics/Universal Bridge  Arms=3  SnubberResistance=1e6  SnubberCapacitance=inf  Device=IGBT / Diodes  Ron=1e-4  Lon=0  ForwardVoltages="[  0  0  ]"  ForwardVoltage=0  GTOparameters=[ 10e-6 , 20e-6 ]  IGBTparameters=[ 1e-6 , 2e-6 ]  Measurements=None  Measurements_2=None  converterType=Rectifier
  A : PMIOPort  Side=Left
  B : PMIOPort  Port=2  Side=Left
  C : PMIOPort  Port=3  Side=Left
  wires:
  Ref/1 -> Universal Bridge/1
  connections:
  Universal Bridge/LConn2 -- B/RConn1
  Universal Bridge/LConn1 -- A/RConn1
  Universal Bridge/LConn3 -- C/RConn1
  Universal Bridge/RConn1 -- DC Voltage Source/RConn1
  Universal Bridge/RConn2 -- DC Voltage Source/LConn1

== system EMT_load/G5/VSC/VSC Model/Phasor ==
  Ref : Inport
  Controlled Current Source : powerlib/Electrical Sources/Controlled Current Source  Initialize=off  Source_Type=AC  Amplitude=0  Phase=0  Frequency=0  Measurements=None
  Controlled Current Source1 : powerlib/Electrical Sources/Controlled Current Source  Initialize=off  Source_Type=AC  Amplitude=0  Phase=0  Frequency=0  Measurements=None
  Controlled Current Source2 : powerlib/Electrical Sources/Controlled Current Source  Initialize=off  Source_Type=AC  Amplitude=0  Phase=0  Frequency=0  Measurements=None
  Demux1 : Demux  Outputs=3
  Ground{1..3,5} (4 alike) : powerlib/Elements/Ground  LConnTagsString=a
  Three-Phase Series RLC Branch : powerlib/Elements/Three-Phase Series RLC Branch  LConnTagsString=A|B|C  RConnTagsString=A|B|C  BranchType=R  Resistance=1e7  Inductance=1e-3  Capacitance=1e-6  Measurements=None
  A : PMIOPort  Side=Left
  B : PMIOPort  Port=2  Side=Left
  C : PMIOPort  Port=3  Side=Left
  wires:
  [c] -> Controlled Current Source2/1
  [b] -> Controlled Current Source1/1
  [a] -> Controlled Current Source/1
  Demux1/3 -> [c]
  Demux1/2 -> [b]
  Demux1/1 -> [a]
  Ref/1 -> Demux1/1
  connections:
  Controlled Current Source/RConn1 -- Ground1/LConn1
  Controlled Current Source1/RConn1 -- Ground2/LConn1
  Controlled Current Source2/RConn1 -- Ground3/LConn1
  A/RConn1 -- Controlled Current Source/LConn1 -- Three-Phase Series RLC Branch/LConn1
  C/RConn1 -- Controlled Current Source2/LConn1 -- Three-Phase Series RLC Branch/LConn3
  Ground5/LConn1 -- Three-Phase Series RLC Branch/RConn2 -- Three-Phase Series RLC Branch/RConn1 -- Three-Phase Series RLC Branch/RConn3
  Controlled Current Source1/LConn1 -- Three-Phase Series RLC Branch/LConn2 -- B/RConn1

== system EMT_load/G6/VSC/VSC Control/Control loops ==
  note: 1) Add Subsystem or Model blocks as valid variant choices.
      | 2) You cannot connect blocks at this level. At simulation, connectivity is automatically
      | determined, based on the active variant and port name matching.
  Pset : Inport
  Qset : Inport  Port=2
  vqd+- : Inport  Port=3
  iqd+- : Inport  Port=4
  freq : Inport  Port=5
  Block : Inport  Port=6
  Phasor I 1st : Subsystem  VariantControl=Phasor_I_1st
  Phasor I ref : Subsystem  VariantControl=Phasor_I_ref
  Phasor PQ 1st : Subsystem  VariantControl=Phasor_PQ
  "SW, EMT AVG, Phasor Quasi-EMT" : Subsystem  VariantControl=EMT_and_QEMT
  vqd+-ref : Outport
  iqd+-ref : Outport  Port=2
  m : Outport  Port=3

== system EMT_load/G6/VSC/VSC Control/Measurements ==
  note: 1) Add Subsystem or Model blocks as valid variant choices.
      | 2) You cannot connect blocks at this level. At simulation, connectivity is automatically
      | determined, based on the active variant and port name matching.
  Vabc : Inport
  Iabc : Inport  Port=2
  EMT : Subsystem  VariantControl=EMT
  Phasor : Subsystem  VariantControl=Phasor
  vqd+- : Outport
  iqd+- : Outport  Port=2
  freq : Outport  Port=3
  theta : Outport  Port=4
  PQabc : Outport  Port=5

== system EMT_load/G6/VSC/VSC Control/Modulation ==
  note: 1) Add Subsystem or Model blocks as valid variant choices.
      | 2) You cannot connect blocks at this level. At simulation, connectivity is automatically
      | determined, based on the active variant and port name matching.
  vqd+- : Inport
  vqd+-* : Inport  Port=2
  iqd+-* : Inport  Port=3
  theta : Inport  Port=4
  EMT AVG : Subsystem  VariantControl=EMT_AVG
  EMT Switching : Subsystem  VariantControl=EMT_SW
  Phasor I and Phasor PQ : Subsystem  VariantControl=Phasor_I_and_PQ
  Phasor Quasi-EMT : Subsystem  VariantControl=Phasor_QEMT
  Ref : Outport

== system EMT_load/G6/VSC/VSC Model/EMT AVG ==
  Ref : Inport
  Controlled Voltage Source3 : spsControlledVoltageSourceLib/Controlled Voltage Source  Initialize=off  Source_Type=AC  Amplitude=Vhvpk  Phase=0  Frequency=fg  Measurements=None
  Controlled Voltage Source4 : spsControlledVoltageSourceLib/Controlled Voltage Source  Initialize=off  Source_Type=AC  Amplitude=Vhvpk  Phase=-2*pi/3  Frequency=fg  Measurements=None
  Controlled Voltage Source5 : spsControlledVoltageSourceLib/Controlled Voltage Source  Initialize=off  Source_Type=AC  Amplitude=Vhvpk  Phase=-4*pi/3  Frequency=fg  Measurements=None
  Demux1 : Demux  Outputs=3
  Ground : spsGroundLib/Ground  LConnTagsString=a
  Ground4 : spsGroundLib/Ground  LConnTagsString=a
  Ground5 : spsGroundLib/Ground  LConnTagsString=a
  A : PMIOPort  Side=Left
  B : PMIOPort  Port=2  Side=Left
  C : PMIOPort  Port=3  Side=Left
  wires:
  Ref/1 -> Demux1/1
  Demux1/1 -> Controlled Voltage Source3/1
  Demux1/2 -> Controlled Voltage Source4/1
  Demux1/3 -> Controlled Voltage Source5/1
  connections:
  Controlled Voltage Source3/RConn1 -- A/RConn1
  Controlled Voltage Source4/RConn1 -- B/RConn1
  Controlled Voltage Source5/RConn1 -- C/RConn1
  Ground/LConn1 -- Controlled Voltage Source3/LConn1
  Ground4/LConn1 -- Controlled Voltage Source4/LConn1
  Ground5/LConn1 -- Controlled Voltage Source5/LConn1

== system EMT_load/G6/VSC/VSC Model/EMT SW ==
  Ref : Inport
  DC Voltage Source : spsDCVoltageSourceLib/DC Voltage Source  Amplitude=Vdc  Measurements=None
  Universal Bridge : spsUniversalBridgeLib/Universal Bridge  Arms=3  SnubberResistance=1e6  SnubberCapacitance=inf  Device=IGBT / Diodes  Ron=1e-4  Lon=0  ForwardVoltages="[  0  0  ]"  ForwardVoltage=0  GTOparameters=[ 10e-6 , 20e-6 ]  IGBTparameters=[ 1e-6 , 2e-6 ]  Measurements=None  Measurements_2=None  converterType=Rectifier
  A : PMIOPort  Side=Left
  B : PMIOPort  Port=2  Side=Left
  C : PMIOPort  Port=3  Side=Left
  wires:
  Ref/1 -> Universal Bridge/1
  connections:
  Universal Bridge/LConn2 -- B/RConn1
  Universal Bridge/LConn1 -- A/RConn1
  Universal Bridge/LConn3 -- C/RConn1
  Universal Bridge/RConn1 -- DC Voltage Source/RConn1
  Universal Bridge/RConn2 -- DC Voltage Source/LConn1

== system EMT_load/G6/VSC/VSC Model/Phasor ==
  Ref : Inport
  Controlled Current Source : spsControlledCurrentSourceLib/Controlled Current Source  Initialize=off  Source_Type=AC  Amplitude=0  Phase=0  Frequency=0  Measurements=None
  Controlled Current Source1 : spsControlledCurrentSourceLib/Controlled Current Source  Initialize=off  Source_Type=AC  Amplitude=0  Phase=0  Frequency=0  Measurements=None
  Controlled Current Source2 : spsControlledCurrentSourceLib/Controlled Current Source  Initialize=off  Source_Type=AC  Amplitude=0  Phase=0  Frequency=0  Measurements=None
  Demux1 : Demux  Outputs=3
  Ground{1..3,5} (4 alike) : spsGroundLib/Ground  LConnTagsString=a
  Three-Phase Series RLC Branch : spsThreePhaseSeriesRLCBranchLib/Three-Phase Series RLC Branch  LConnTagsString=A|B|C  RConnTagsString=A|B|C  BranchType=R  Resistance=1e7  Inductance=1e-3  Capacitance=1e-6  Measurements=None
  A : PMIOPort  Side=Left
  B : PMIOPort  Port=2  Side=Left
  C : PMIOPort  Port=3  Side=Left
  wires:
  [c] -> Controlled Current Source2/1
  [b] -> Controlled Current Source1/1
  [a] -> Controlled Current Source/1
  Demux1/3 -> [c]
  Demux1/2 -> [b]
  Demux1/1 -> [a]
  Ref/1 -> Demux1/1
  connections:
  Controlled Current Source/RConn1 -- Ground1/LConn1
  Controlled Current Source1/RConn1 -- Ground2/LConn1
  Controlled Current Source2/RConn1 -- Ground3/LConn1
  A/RConn1 -- Controlled Current Source/LConn1 -- Three-Phase Series RLC Branch/LConn1
  C/RConn1 -- Controlled Current Source2/LConn1 -- Three-Phase Series RLC Branch/LConn3
  Ground5/LConn1 -- Three-Phase Series RLC Branch/RConn2 -- Three-Phase Series RLC Branch/RConn1 -- Three-Phase Series RLC Branch/RConn3
  Controlled Current Source1/LConn1 -- Three-Phase Series RLC Branch/LConn2 -- B/RConn1

== system EMT_load/G6s/Exciter System/SEXS/1st ord transfer fcn windup limiter ==
  note: First order transfer function with windup limiter (non-saturated output)
  In1 : Inport
  Compare To Constant : simulink/Logic and Bit Operations/Compare To Constant  relop=<=  const=Vmax  OutDataTypeStr=boolean
  Compare To Constant1 : simulink/Logic and Bit Operations/Compare To Constant  relop=>=  const=Vmin  OutDataTypeStr=boolean
  OR : Logic  Operator=OR  IconShape=distinctive  AllPortsSameDT=off  OutDataTypeStr=boolean
  Sample and Hold1 : spsSampleandHoldLib/Sample and Hold  ic=0  Ts=0
      settings: LibrarySourceBlock=|
      | sps_lib/Control/Sample and
      | Hold
  Saturation1 : Saturate  UpperLimit=Vmax  LowerLimit=Vmin
  Transfer Fcn (with initial outputs)2 : simulink_extras/Additional Linear/Transfer Fcn (with initial outputs)  N=[Gain]  D=[tau 1]  Y0=y0  U0=y0/Gain
  Out1 : Outport
  wires:
  Sample and Hold1/1 -> Transfer Fcn (with initial outputs)2/1
  Transfer Fcn (with initial outputs)2/1 -> Saturation1/1, Compare To Constant1/1, Compare To Constant/1
  In1/1 -> Sample and Hold1/1
  Compare To Constant/1 -> OR/1
  Compare To Constant1/1 -> OR/2
  OR/1 -> Sample and Hold1/2
  Saturation1/1 -> Out1/1

== system EMT_load/G7/Exciter System/SEXS/1st ord transfer fcn windup limiter ==
  note: First order transfer function with windup limiter (non-saturated output)
  In1 : Inport
  Compare To Constant : simulink/Logic and Bit Operations/Compare To Constant  relop=<=  const=Vmax  OutDataTypeStr=boolean
  Compare To Constant1 : simulink/Logic and Bit Operations/Compare To Constant  relop=>=  const=Vmin  OutDataTypeStr=boolean
  OR : Logic  Operator=OR  IconShape=distinctive  AllPortsSameDT=off  OutDataTypeStr=boolean
  Sample and Hold1 : spsSampleandHoldLib/Sample and Hold  ic=0  Ts=0
      settings: LibrarySourceBlock=|
      | sps_lib/Control/Sample and
      | Hold
  Saturation1 : Saturate  UpperLimit=Vmax  LowerLimit=Vmin
  Transfer Fcn (with initial outputs)2 : simulink_extras/Additional Linear/Transfer Fcn (with initial outputs)  N=[Gain]  D=[tau 1]  Y0=y0  U0=y0/Gain
  Out1 : Outport
  wires:
  Sample and Hold1/1 -> Transfer Fcn (with initial outputs)2/1
  Transfer Fcn (with initial outputs)2/1 -> Saturation1/1, Compare To Constant1/1, Compare To Constant/1
  In1/1 -> Sample and Hold1/1
  Compare To Constant/1 -> OR/1
  Compare To Constant1/1 -> OR/2
  OR/1 -> Sample and Hold1/2
  Saturation1/1 -> Out1/1

== system EMT_load/G2/VSC/VSC Control/Control loops/Phasor I 1st ==
  Pset : Inport
  Qset : Inport  Port=2
  vqd+- : Inport  Port=3
  iqd+- : Inport  Port=4
  freq : Inport  Port=5
  Block : Inport  Port=6
  Inner-loop : Subsystem
  Mux : Mux
  Outer-loop : Subsystem
      settings: PortSchema="{\"entries\":[{\"content\":{\"sides\":[{\"content\":{\"connectorIds\":[\"In1\",\"In2\",\"In3\",\"In4\",\"In5\"]},\"type\":\"ConnectorPlacement.EquallySpacedRectSide\",\"uuid\":\"9a334ab0-c6a2-41fb-a6ec-750715335523\"},{\"content\":{\"connectorIds\":[\"Out1\",\"Out2\",\"Out3\",\"Out4\",\"Out5\"],\"side\":\"RIGHT\"},\"type\":\"ConnectorPlacement.EquallySpacedRectSide\",\"uuid\":\"d3309230-0110-441f-b944-3d5d4312a42e\"},{\"content\":{\"connectorIds\":[\"In6\"],\"side\":\"TOP\"},\"type\":\"ConnectorPlacement.EquallySpacedRectSide\",\"uuid\":\"012603a1-4678-4ae1-91f6-3e17a1c8130b\"}]},\"type\":\"ConnectorPlacement.EquallySpacedConnector\",\"uuid\":\"299866d5-057c-44fe-b725-733ff7b8fc12\"}],\"packageUris\":[\"http://schema.mathworks.com/mf0/Connector/19700101\"],\"version\":\"1.0\"}"
  iqd+-ref : Outport
  m : Outport  Port=2
  wires:
  Outer-loop/4(id-*) -> Inner-loop/4(id-*)
  Outer-loop/3(iq-*) -> Inner-loop/3(iq-*)
  Outer-loop/2(id+*) -> Inner-loop/2(id+*)
  Outer-loop/1(iq+*) -> Inner-loop/1(iq+*)
  Block/1 -> Outer-loop/6(Blk)
  vqd+-/1 -> Outer-loop/3(vqd+-)
  freq/1 -> Outer-loop/5(freq)
  iqd+-/1 -> Outer-loop/4(iqd+-)
  Inner-loop/2(id+ref) -> Mux/2
  Pset/1 -> Outer-loop/1(Pset)
  Outer-loop/5(m) -> m/1
  Qset/1 -> Outer-loop/2(Qset)
  Mux/1 -> iqd+-ref/1
  Inner-loop/3(iq-ref) -> Mux/3
  Inner-loop/1(iq+ref) -> Mux/1
  Inner-loop/4(id-ref) -> Mux/4

== system EMT_load/G2/VSC/VSC Control/Control loops/Phasor I ref ==
  Pset : Inport
  Qset : Inport  Port=2
  vqd+- : Inport  Port=3
  iqd+- : Inport  Port=4
  freq : Inport  Port=5
  Block : Inport  Port=6
  Mux : Mux
  Outer-loop : Subsystem
      settings: PortSchema="{\"entries\":[{\"content\":{\"sides\":[{\"content\":{\"connectorIds\":[\"In1\",\"In2\",\"In3\",\"In4\",\"In5\"]},\"type\":\"ConnectorPlacement.EquallySpacedRectSide\",\"uuid\":\"9a334ab0-c6a2-41fb-a6ec-750715335523\"},{\"content\":{\"connectorIds\":[\"Out1\",\"Out2\",\"Out3\",\"Out4\",\"Out5\"],\"side\":\"RIGHT\"},\"type\":\"ConnectorPlacement.EquallySpacedRectSide\",\"uuid\":\"d3309230-0110-441f-b944-3d5d4312a42e\"},{\"content\":{\"connectorIds\":[\"In6\"],\"side\":\"TOP\"},\"type\":\"ConnectorPlacement.EquallySpacedRectSide\",\"uuid\":\"012603a1-4678-4ae1-91f6-3e17a1c8130b\"}]},\"type\":\"ConnectorPlacement.EquallySpacedConnector\",\"uuid\":\"299866d5-057c-44fe-b725-733ff7b8fc12\"}],\"packageUris\":[\"http://schema.mathworks.com/mf0/Connector/19700101\"],\"version\":\"1.0\"}"
  iqd+-ref : Outport
  m : Outport  Port=2
  wires:
  Outer-loop/4(id-*) -> Mux/4
  Outer-loop/1(iq+*) -> Mux/1
  Outer-loop/3(iq-*) -> Mux/3
  Mux/1 -> iqd+-ref/1
  Qset/1 -> Outer-loop/2(Qset)
  Outer-loop/5(m) -> m/1
  Pset/1 -> Outer-loop/1(Pset)
  Outer-loop/2(id+*) -> Mux/2
  iqd+-/1 -> Outer-loop/4(iqd+-)
  freq/1 -> Outer-loop/5(freq)
  vqd+-/1 -> Outer-loop/3(vqd+-)
  Block/1 -> Outer-loop/6(Blk)

== system EMT_load/G2/VSC/VSC Control/Control loops/Phasor PQ 1st ==
  Pset : Inport
  Qset : Inport  Port=2
  vqd+- : Inport  Port=3
  iqd+- : Inport  Port=4
  freq : Inport  Port=5
  Block : Inport  Port=6
  Mux : Mux
  Outer-loop : Subsystem
      settings: PortSchema="{\"entries\":[{\"content\":{\"sides\":[{\"content\":{\"connectorIds\":[\"In1\",\"In2\",\"In3\",\"In4\",\"In5\"]},\"type\":\"ConnectorPlacement.EquallySpacedRectSide\",\"uuid\":\"9a334ab0-c6a2-41fb-a6ec-750715335523\"},{\"content\":{\"connectorIds\":[\"Out1\",\"Out2\",\"Out3\",\"Out4\",\"Out5\"],\"side\":\"RIGHT\"},\"type\":\"ConnectorPlacement.EquallySpacedRectSide\",\"uuid\":\"d3309230-0110-441f-b944-3d5d4312a42e\"},{\"content\":{\"connectorIds\":[\"In6\"],\"side\":\"TOP\"},\"type\":\"ConnectorPlacement.EquallySpacedRectSide\",\"uuid\":\"012603a1-4678-4ae1-91f6-3e17a1c8130b\"}]},\"type\":\"ConnectorPlacement.EquallySpacedConnector\",\"uuid\":\"299866d5-057c-44fe-b725-733ff7b8fc12\"}],\"packageUris\":[\"http://schema.mathworks.com/mf0/Connector/19700101\"],\"version\":\"1.0\"}"
  iqd+-ref : Outport
  m : Outport  Port=2
  wires:
  Block/1 -> Outer-loop/6(Blk)
  vqd+-/1 -> Outer-loop/3(vqd+-)
  freq/1 -> Outer-loop/5(freq)
  iqd+-/1 -> Outer-loop/4(iqd+-)
  Outer-loop/2(id+*) -> Mux/2
  Pset/1 -> Outer-loop/1(Pset)
  Outer-loop/5(m) -> m/1
  Qset/1 -> Outer-loop/2(Qset)
  Mux/1 -> iqd+-ref/1
  Outer-loop/3(iq-*) -> Mux/3
  Outer-loop/1(iq+*) -> Mux/1
  Outer-loop/4(id-*) -> Mux/4
